simulink model "DC_motor_state_feedback"  (Simulink 8.9)
settings: Solver=VariableStepAuto  StartTime=0.0  StopTime=10.0  RelTol=1e-3
values from neighbouring files (symbols this model uses):
  A = diag([-1 -2, -100, -200])    [HW9.m]    (also in extra_credit.m = -5; systems_matlab_examples.m = [1 2; 3, 1]; systems_p1_guide.m = [-1 0 ; 0 -2])
  B = [1;1;1;1]    [HW9.m]    (also in extra_credit.m = 2; systems_matlab_examples.m = [ 0; 1]; systems_p1_guide.m = [1;1])
  C = [1 1 0.5 0.5]    [HW9.m]    (also in extra_credit.m = 1; systems_matlab_examples.m = [1 1]; systems_p1_guide.m = eye(2))
undefined symbols (not defined in the file or in its folder): IC, K
settings Model: Creator=Merc  LastModifiedBy=Merc
settings DataIOCC: LimitDataPoints=off  SaveFormat=Dataset  SignalLoggingSaveFormat=Dataset
settings OptimizationCC: LifeSpan=auto
settings DebuggingCC: UnderspecifiedInitializationDetection=Simplified  MergeDetectMultiDrivingBlocksExec=error  FcnCallInpInsideContextMsg=error  StateNameClashWarn=none  SFUnexpectedBacktrackingDiag=error  SFNoUnconditionalDefaultTransitionDiag=error  SFExecutionAtInitializationDiag=warning
settings HardwareCC: ProdBitPerPointer=64  ProdBitPerSizeT=64  ProdBitPerPtrDiffT=64  ProdLargestAtomicFloat=Float  ProdIntDivRoundTo=Zero  ProdEndianess=LittleEndian  ProdWordSize=64  ProdHWDeviceType=Intel->x86-64 (Windows64)
settings ModelReferenceCC: PropagateSignalLabelsOutOfModel=on
settings GRTTargetCC: TargetLangStandard=C99 (ISO)  GeneratePreprocessorConditionals=Use local settings  CombineOutputUpdateFcns=on  GRTInterface=off
settings ConfigComp: CovMetricSettings=dwe  CovHtmlReporting=off  CovSaveCumulativeToWorkspaceVar=off  CovSaveSingleToWorkspaceVar=off  CovExternalEMLEnable=on

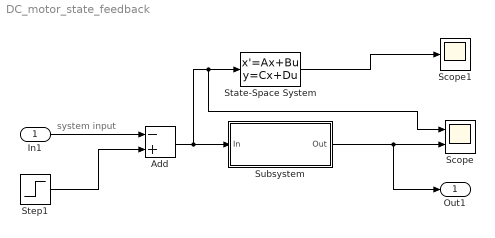
== system DC_motor_state_feedback ==
  note: system input
  In1 : Inport
  Add : Sum  Inputs=-+
  Scope : Scope  NumInputPorts=2
  Scope1 : Scope
  State-Space System : StateSpace  A=A  B=B  C=eye(2)  D=[0;0]  X0=IC  ContinuousStateAttributes='openloop'
  Step1 : Step  Time=0.3  After=10  SampleTime=0
  Subsystem : Subsystem
  Out1 : Outport
  wires:
  In1/1 -> Add/1
  Step1/1 -> Add/2
  Add/1 -> Scope/1, State-Space System/1, Subsystem/1(In)
  Subsystem/1("Out ") -> Out1/1, Scope/2
  State-Space System/1 -> Scope1/1

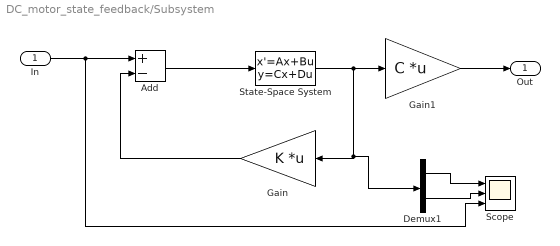
== system DC_motor_state_feedback/Subsystem ==
  In : Inport
  Add : Sum  Inputs=+-
  Demux1 : Demux  Outputs=2
  Gain : Gain  Gain=K  Multiplication=Matrix(K*u) (u vector)
  Gain1 : Gain  Gain=C  Multiplication=Matrix(K*u) (u vector)
  Scope : Scope  NumInputPorts=3
  State-Space System : StateSpace  A=A  B=B  C=eye(2)  D=[0;0]  X0=IC
  "Out " : Outport
  wires:
  In/1 -> Scope/3, Add/1
  Add/1 -> State-Space System/1
  State-Space System/1 -> Demux1/1, Gain/1, Gain1/1
  Gain1/1 -> "Out "/1
  Gain/1 -> Add/2
  Demux1/1 -> Scope/1
  Demux1/2 -> Scope/2
